simulink model "IEEE5Bus"  (R2020a)
settings: Solver=ode23tb  StartTime=0.0  StopTime=20/60  RelTol=1e-3  EnableMultiTasking=on
libraries: powerlib x47, simulink x1
(part 2 of 2)

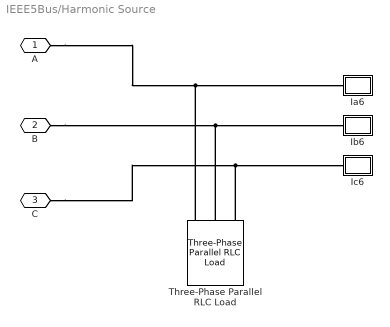
== system IEEE5Bus/Harmonic Source ==
  Ia6 : Subsystem
  Ib6 : Subsystem
  Ic6 : Subsystem
  Three-Phase Parallel RLC Load : powerlib/Elements/Three-Phase Parallel RLC Load  LConnTagsString=A|B|C  Configuration=Y (grounded)  NominalVoltage=220e3  Vabc=[1e3 1e3 1e3]  Vabcp=[1e3 1e3 1e3]  NominalFrequency=60  UnbalancedPower=off  ActivePower=745e3  InductivePower=245e3  CapacitivePower=245e3  Pabc=[10e3 9e3 11e3]  QLabc=[100 90 110]  QCabc=[100 90 110]  Pabcp=[10e3 9e3 11e3]  QLabcp=[100 90 110]  QCabcp=[100 90 110]  Measurements=None  LoadType=constant Z
  A : PMIOPort  Side=Right
  B : PMIOPort  Port=2  Side=Right
  C : PMIOPort  Port=3  Side=Right
  connections:
  B/RConn1 -- Three-Phase Parallel RLC Load/LConn2 -- Ib6/RConn1
  C/RConn1 -- Three-Phase Parallel RLC Load/LConn3 -- Ic6/RConn1
  A/RConn1 -- Three-Phase Parallel RLC Load/LConn1 -- Ia6/RConn1

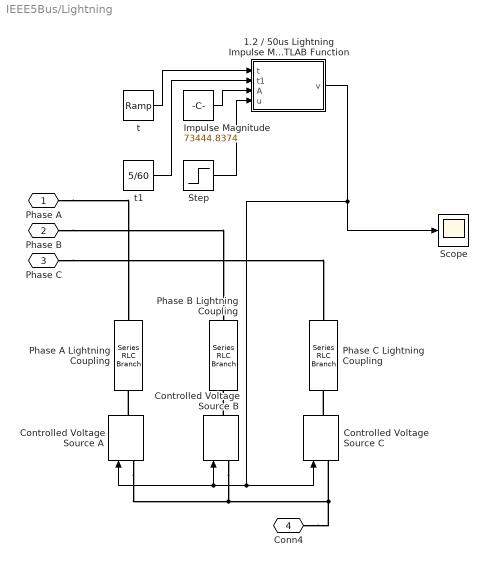
== system IEEE5Bus/Lightning ==
  1.2 / 50us Lightning Impulse MATLAB Function : MATLAB Function  TreatAsAtomicUnit=on
  Controlled Voltage Source C : powerlib/Electrical Sources/Controlled Voltage Source  Initialize=on  Source_Type=DC  Amplitude=0  Phase=0  Frequency=0  Measurements=None
  Controlled Voltage Source A : powerlib/Electrical Sources/Controlled Voltage Source  Initialize=on  Source_Type=DC  Amplitude=0  Phase=0  Frequency=0  Measurements=None
  Controlled Voltage Source B : powerlib/Electrical Sources/Controlled Voltage Source  Initialize=on  Source_Type=DC  Amplitude=0  Phase=0  Frequency=0  Measurements=None
  Impulse Magnitude : Constant  Value=73444.8374  SampleTime=5e-6
  Phase A Lightning Coupling : powerlib/Elements/Series RLC Branch  LConnTagsString=__new0  RConnTagsString=__new0  BranchType=RC  Resistance=1  Inductance=1.5e-1  SetiL0=off  InitialCurrent=0  Capacitance=3e-6  Setx0=off  InitialVoltage=0  Measurements=None
  Phase B Lightning Coupling : powerlib/Elements/Series RLC Branch  LConnTagsString=__new0  RConnTagsString=__new0  BranchType=RC  Resistance=1  Inductance=1.5e-1  SetiL0=off  InitialCurrent=0  Capacitance=3e-6  Setx0=off  InitialVoltage=0  Measurements=None
  Phase C Lightning Coupling : powerlib/Elements/Series RLC Branch  LConnTagsString=__new0  RConnTagsString=__new0  BranchType=RC  Resistance=1  Inductance=1.5e-1  SetiL0=off  InitialCurrent=0  Capacitance=3e-6  Setx0=off  InitialVoltage=0  Measurements=None
  Scope : Scope
  Step : Step  Time=5/60  SampleTime=0
  t : simulink/Sources/Ramp  slope=1  start=0  InitialOutput=0
  t1 : Constant  Value=5/60
  Phase A : PMIOPort  Side=Left
  Phase B : PMIOPort  Port=2  Side=Left
  Phase C : PMIOPort  Port=3  Side=Left
  Conn4 : PMIOPort  Port=4  Side=Left
  wires:
  Impulse Magnitude/1 -> 1.2 / 50us Lightning Impulse MATLAB Function/3(A)
  t/1 -> 1.2 / 50us Lightning Impulse MATLAB Function/1(t)
  1.2 / 50us Lightning Impulse MATLAB Function/1(v) -> Scope/1, Controlled Voltage Source A/1, Controlled Voltage Source B/1, Controlled Voltage Source C/1
  t1/1 -> 1.2 / 50us Lightning Impulse MATLAB Function/2(t1)
  Step/1 -> 1.2 / 50us Lightning Impulse MATLAB Function/4(u)
  connections:
  Phase B/RConn1 -- Phase B Lightning Coupling/LConn1
  Phase C/RConn1 -- Phase C Lightning Coupling/LConn1
  Controlled Voltage Source B/LConn1 -- Conn4/RConn1 -- Controlled Voltage Source C/LConn1 -- Controlled Voltage Source A/LConn1
  Controlled Voltage Source C/RConn1 -- Phase C Lightning Coupling/RConn1
  Phase A/RConn1 -- Phase A Lightning Coupling/LConn1
  Controlled Voltage Source A/RConn1 -- Phase A Lightning Coupling/RConn1
  Controlled Voltage Source B/RConn1 -- Phase B Lightning Coupling/RConn1

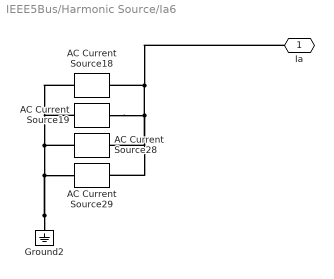
== system IEEE5Bus/Harmonic Source/Ia6 ==
  AC Current Source18 : powerlib/Electrical Sources/AC Current Source  Amplitude=18.152/2  Phase=30.64  Frequency=300  SampleTime=5e-6  Measurements=None
      settings: SourceProductBaseCode=PS
  AC Current Source19 : powerlib/Electrical Sources/AC Current Source  Amplitude=20.996/2  Phase=16.67  Frequency=420  SampleTime=5e-6  Measurements=None
      settings: SourceProductBaseCode=PS
  AC Current Source28 : powerlib/Electrical Sources/AC Current Source  Amplitude=6.307  Phase=-205.35  Frequency=660  SampleTime=5e-6  Measurements=None
      settings: SourceProductBaseCode=PS
  AC Current Source29 : powerlib/Electrical Sources/AC Current Source  Amplitude=5.554  Phase=-226.36  Frequency=720  SampleTime=5e-6  Measurements=None
      settings: SourceProductBaseCode=PS
  Ground2 : powerlib/Elements/Ground  LConnTagsString=a
  Ia : PMIOPort  Side=Right
  connections:
  Ground2/LConn1 -- AC Current Source18/LConn1 -- AC Current Source19/LConn1 -- AC Current Source28/LConn1 -- AC Current Source29/LConn1
  Ia/RConn1 -- AC Current Source18/RConn1 -- AC Current Source19/RConn1 -- AC Current Source28/RConn1 -- AC Current Source29/RConn1

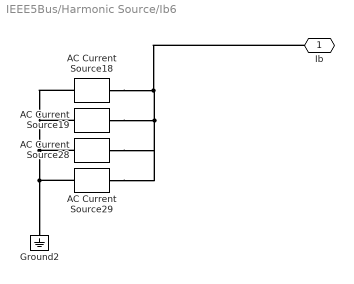
== system IEEE5Bus/Harmonic Source/Ib6 ==
  AC Current Source18 : powerlib/Electrical Sources/AC Current Source  Amplitude=18.152/2  Phase=30.64+120  Frequency=300  SampleTime=5e-6  Measurements=None
      settings: SourceProductBaseCode=PS
  AC Current Source19 : powerlib/Electrical Sources/AC Current Source  Amplitude=20.996/2  Phase=16.67-120  Frequency=420  SampleTime=5e-6  Measurements=None
      settings: SourceProductBaseCode=PS
  AC Current Source28 : powerlib/Electrical Sources/AC Current Source  Amplitude=6.307  Phase=-205.35+120  Frequency=660  SampleTime=5e-6  Measurements=None
      settings: SourceProductBaseCode=PS
  AC Current Source29 : powerlib/Electrical Sources/AC Current Source  Amplitude=5.554  Phase=-226.36-120  Frequency=720  SampleTime=5e-6  Measurements=None
      settings: SourceProductBaseCode=PS
  Ground2 : powerlib/Elements/Ground  LConnTagsString=a
  Ib : PMIOPort  Side=Right
  connections:
  AC Current Source29/RConn1 -- AC Current Source28/RConn1 -- AC Current Source19/RConn1 -- AC Current Source18/RConn1 -- Ib/RConn1
  AC Current Source19/LConn1 -- AC Current Source18/LConn1 -- AC Current Source28/LConn1 -- AC Current Source29/LConn1 -- Ground2/LConn1

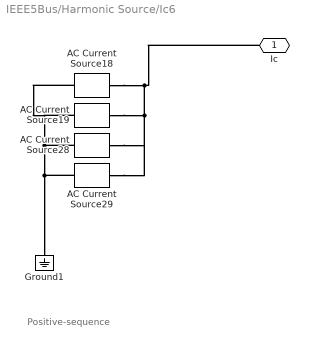
== system IEEE5Bus/Harmonic Source/Ic6 ==
  note: Positive-sequence
  AC Current Source18 : powerlib/Electrical Sources/AC Current Source  Amplitude=18.152/2  Phase=30.64-120  Frequency=300  SampleTime=5e-6  Measurements=None
      settings: SourceProductBaseCode=PS
  AC Current Source19 : powerlib/Electrical Sources/AC Current Source  Amplitude=20.996/2  Phase=16.67+120  Frequency=420  SampleTime=5e-6  Measurements=None
      settings: SourceProductBaseCode=PS
  AC Current Source28 : powerlib/Electrical Sources/AC Current Source  Amplitude=6.307  Phase=-205.35-120  Frequency=660  SampleTime=5e-6  Measurements=None
      settings: SourceProductBaseCode=PS
  AC Current Source29 : powerlib/Electrical Sources/AC Current Source  Amplitude=5.554  Phase=-226.36+120  Frequency=720  SampleTime=5e-6  Measurements=None
      settings: SourceProductBaseCode=PS
  Ground1 : powerlib/Elements/Ground  LConnTagsString=a
  Ic : PMIOPort  Side=Right
  connections:
  AC Current Source19/LConn1 -- AC Current Source18/LConn1 -- AC Current Source28/LConn1 -- AC Current Source29/LConn1 -- Ground1/LConn1
  Ic/RConn1 -- AC Current Source18/RConn1 -- AC Current Source19/RConn1 -- AC Current Source29/RConn1 -- AC Current Source28/RConn1

== matlab function IEEE5Bus/Lightning/1.2 // 50us Lightning Impulse MATLAB Function ==
  data: t input; t1 input; A input; v output; u input
function v = fcn(t,t1,A,u)
alpha=14000;
v = A*exp(-alpha*abs(t-t1))*u;
